simulink model "Fault_Below20_5Steps_NoCounter"  (R2025a)
settings: Solver=VariableStepAuto  StartTime=0.0  StopTime=10.0  RelTol=1e-3
libraries: simulink x4
settings Model: Creator=mahij  LastModifiedBy=mahij

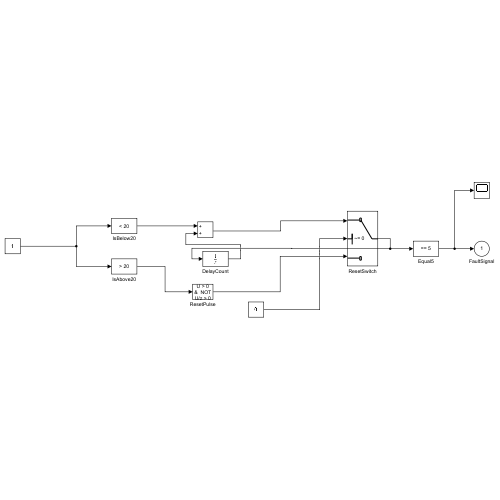
[thumbnail: Simulink's stored preview of the top-level diagram]
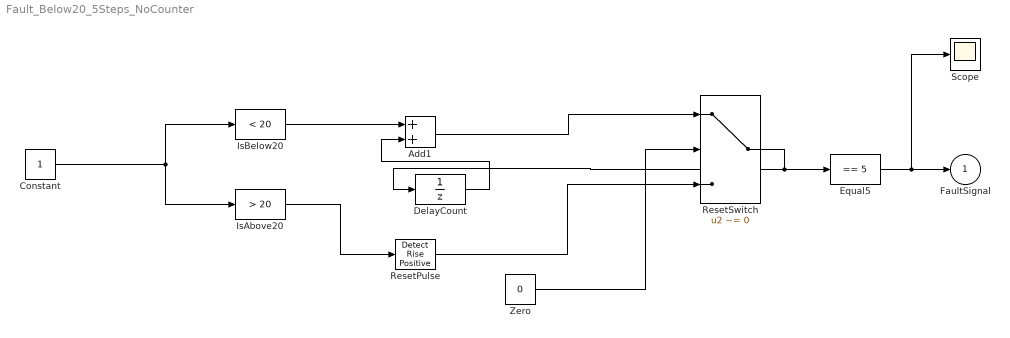
== system Fault_Below20_5Steps_NoCounter ==
  Add1 : Sum
  Constant : Constant
  DelayCount : UnitDelay  SampleTime=-1  HasFrameUpgradeWarning=on
  Equal5 : simulink/Logic and Bit Operations/Compare To Constant  relop===  const=5  OutDataTypeStr=boolean
  IsAbove20 : simulink/Logic and Bit Operations/Compare To Constant  relop=>  const=20  OutDataTypeStr=boolean
  IsBelow20 : simulink/Logic and Bit Operations/Compare To Constant  relop=<  const=20  OutDataTypeStr=boolean
  ResetPulse : simulink/Logic and Bit Operations/Detect Rise Positive  vinit=0  OutDataTypeStr=boolean
  ResetSwitch : Switch  Criteria=u2 ~= 0  Threshold=0.5  SaturateOnIntegerOverflow=off  InputSameDT=off
  Scope : Scope
  Zero : Constant  Value=0
  FaultSignal : Outport
  wires:
  Constant/1 -> IsBelow20/1, IsAbove20/1
  IsAbove20/1 -> ResetPulse/1
  IsBelow20/1 -> Add1/1
  DelayCount/1 -> Add1/2
  Add1/1 -> ResetSwitch/1
  Zero/1 -> ResetSwitch/2
  ResetPulse/1 -> ResetSwitch/3
  ResetSwitch/1 -> DelayCount/1, Equal5/1
  Equal5/1 -> Scope/1, FaultSignal/1
